simulink model "IFFT64K_2D"  (R2023b)
settings: Solver=VariableStepAuto  StartTime=0.0  StopTime=simtime  RelTol=1e-3
PostLoadFcn:
  | samp_rate = 2e9;
  | fft_sz = 65536;
  | chirp_rate = 200e6 / 1e-3;
  | tone_freq = 20e6;
  | input_bits = 12;
  | align_delay = 3 * fft_sz;
  | buff_init = complex(int32(zeros(256,1)));
  | NSTREAM = 5;
  | simtime = 2.5e-4;
undefined symbols (not defined in the file): S, vsva2197, xcvc1902
libraries: aieBasic x30, aieUtilities x15, hlsBasic x1, dspxfrm3 x1, dspsrcs4 x1, vmcUtilities x1
(part 1 of 2)
settings Model: Creator=rbuz  LastModifiedBy=robg
settings DebuggingCC: UnconnectedInputMsg=warning  UnconnectedOutputMsg=warning  UnconnectedLineMsg=warning
settings ModelReferenceCC: EnableRefExpFcnMdlSchedulingChecks=on
settings RTWCC: DLArmComputeVersion=19.05

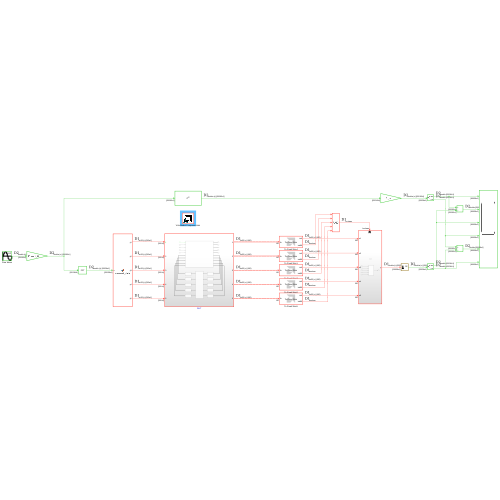
[thumbnail: Simulink's stored preview of the top-level diagram]
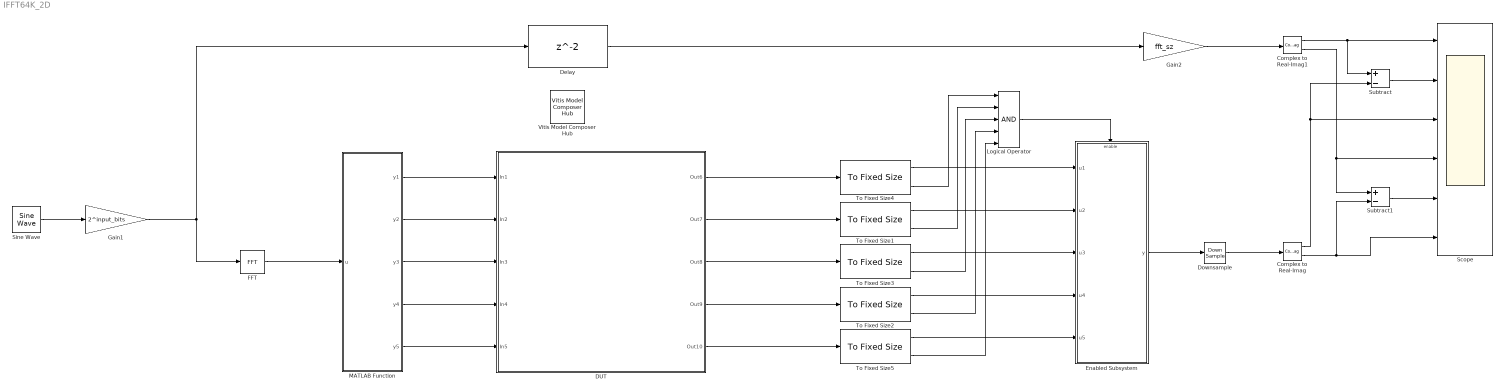
== system IFFT64K_2D ==
  Complex to Real-Imag : ComplexToRealImag
  Complex to Real-Imag1 : ComplexToRealImag
  DUT : Subsystem
  Delay : Delay
  Downsample : DownSample  N=52  RateOptions=Allow multirate processing
  Enabled Subsystem : Subsystem  TreatAsAtomicUnit=on
  FFT : dspxfrm3/FFT  FFTImplementation=Auto  CompMethod=Table lookup  TableOpt=NEW  TableOptActive=Speed  BitRevOrder=off  Normalize=off  InheritFFTLength=off  FFTLength=fft_sz  WrapInput=off  roundingMode=Floor  overflowMode=off  firstCoeffDataTypeStr=Inherit: Same word length as input  firstCoeffLastDataTypeStr=Inherit: Same word length as input  outputMin=[]  outputMax=[]
  Gain1 : Gain  Gain=2^input_bits
  Gain2 : Gain  Gain=fft_sz
  Logical Operator : Logic  Inputs=5  AllPortsSameDT=off  OutDataTypeStr=boolean
  MATLAB Function : MATLAB Function  TreatAsAtomicUnit=on  SystemSampleTime=fft_sz / (52 * samp_rate)
  Scope : Scope  NumInputPorts=6
  Sine Wave : dspsrcs4/Sine Wave  Amplitude=1  Frequency=tone_freq  Phase=0  SampleMode=Discrete  OutComplex=Complex  CompMethod=Trigonometric fcn  TableSize=Speed  SampleTime=1 / samp_rate  SamplesPerFrame=fft_sz  ResetState=Restart at time zero  OutputFrames=off  dataType=double  wordLen=16  udDataType=sfix(16)  fracBitsMode=Best precision  numFracBits=15  OutDataTypeStr=double  LastOutDataTypeStr=double
  Subtract : Sum  Inputs=+-
  Subtract1 : Sum  Inputs=+-
  To Fixed Size{1..5} (5 alike) : aieUtilities/To Fixed Size  Mode=Produce a valid output signal  OutputSize=Inherit: Same as input  CopyMethod=Buffer samples to form output  HasStatusOutput=on
  Vitis Model Composer Hub : vmcUtilities/Vitis Model Composer Hub  Tag=genX  CodeGeneration=off  SubsystemName=DUT  DUTSubsystemName=DUT  CompilationType=VitisCompilation  SubsystemType=DUTNode  ExportTypeV2=Graph Code  AIEArrayConfig=Use entire AIE array  StartColumn=20  NumberOfColumns=10  TargetDirectory=./code  exportDesign=on  analyzeDesign=off  validateDesignOnHw=off  ExportType=Vitis Subsystem  IpVendor=xilinx.com  IpLibrary=hls  IpName=ifft_transpose  IpVersion=1.0  IpHWLanguage=Verilog  AieCompilerOptions={}  AieSimulatorOptions={}  CreateTestbench=off  TestbenchStackSize=10  RunRtlSim=off  RunCSim=off  RunAieSim=on  AieSimTimeout=50000  RunAieSimProfiling=off  LaunchVitisAnalyzer=off  PlotOutput=off  RunX86Sim=off  X86SimTimeout=10  GenHwImage=off  GenLibadfXo=on  GenHwValidationCode=on  PlatformType=Specify Platform  Platform=/proj/xbuilds/SWIP/2024.2_1110_1447/installs/lin64/Vitis/2024.2/base_platforms/xilinx_vck190_base_202420_1/xilinx_vck190_base_202420_1.xpfm  HwSystemType=Baremetal  HwValidationTarget=hw_emu  ProjDevice=Versal VCK190 Evaluation Platform (xcvc1902-vsva2197-2MP-e-S)  ProjDevicePart=xcvc1902-vsva2197-2MP-e-S  AIEType=AIE  SamplePeriod=-1  ClockFrequency=200  DataPathParallelism=1  xilinxfamily=versalaicore  part=xcvc1902  speed=-2MP-e-S  package=vsva2197  directory=./netlist  testbench=off  incr_netlist=off  synthesis_tool=Vivado  clock_wrapper=Clock Enables  dbl_ovrd=According to Block Masks  dcm_input_clock_period=10  sysclk_period=10  simulink_period=1  eval_field=0  IPInfoJsonString="{\"DUTSubsystemName\":\"DUT\",\"HLSKernel\":{\"SubsystemName\":\"ifft_transpose\",\"FpgaClockFreq\":\"200\",\"IPName\":\"ifft_transpose\",\"IPLibrary\":\"hls\",\"TargetDirectory\":\"./code\",\"FreqHz\":\"200000000\",\"KernelFunction\":\"ifft_transpose_wrapper\"},\"SubsystemTag\":\"DUTNode\",\"AIESubsystem\":{\"SubsystemName\":\"AIE\",\"TargetDirectory\":\"./code\",\"AIEArrayConfig\":\"Use entire AIE array\",\"StartColumn\":\"20\",\"NumberOfColumns\":\"10\"}}"  LogFileName=/group/xcoswmktg2/robg/git/vmc_examples/Vitis_Model_Composer/Tutorials/AIE-PL/Export_to_Vitis/code/model_composer.log  NThreads=4  IPConfigFile=/tmp/vmctmp-robg/11175/ipconfig.json
  wires:
  Gain1/1 -> FFT/1, Delay/1
  Sine Wave/1 -> Gain1/1
  FFT/1 -> MATLAB Function/1(u)
  MATLAB Function/1(y1) -> DUT/1(In1)
  To Fixed Size4/1 -> Enabled Subsystem/1(u1)
  Enabled Subsystem/1(y) -> Downsample/1
  Subtract/1 -> Scope/2
  Subtract1/1 -> Scope/5
  Delay/1 -> Gain2/1
  Complex to Real-Imag1/1 -> Scope/1, Subtract/1
  Complex to Real-Imag1/2 -> Scope/4, Subtract1/1
  Complex to Real-Imag/1 -> Scope/3, Subtract/2
  Complex to Real-Imag/2 -> Subtract1/2, Scope/6
  Gain2/1 -> Complex to Real-Imag1/1
  MATLAB Function/2(y2) -> DUT/2(In2)
  MATLAB Function/3(y3) -> DUT/3(In3)
  MATLAB Function/4(y4) -> DUT/4(In4)
  MATLAB Function/5(y5) -> DUT/5(In5)
  To Fixed Size1/1 -> Enabled Subsystem/2(u2)
  To Fixed Size3/1 -> Enabled Subsystem/3(u3)
  To Fixed Size2/1 -> Enabled Subsystem/4(u4)
  To Fixed Size5/1 -> Enabled Subsystem/5(u5)
  Logical Operator/1 -> Enabled Subsystem/Enable
  To Fixed Size4/2 -> Logical Operator/1
  To Fixed Size1/2 -> Logical Operator/2
  To Fixed Size3/2 -> Logical Operator/3
  To Fixed Size2/2 -> Logical Operator/4
  To Fixed Size5/2 -> Logical Operator/5
  DUT/1(Out6) -> To Fixed Size4/1
  DUT/2(Out7) -> To Fixed Size1/1
  DUT/3(Out8) -> To Fixed Size3/1
  DUT/4(Out9) -> To Fixed Size2/1
  DUT/5(Out10) -> To Fixed Size5/1
  Downsample/1 -> Complex to Real-Imag/1

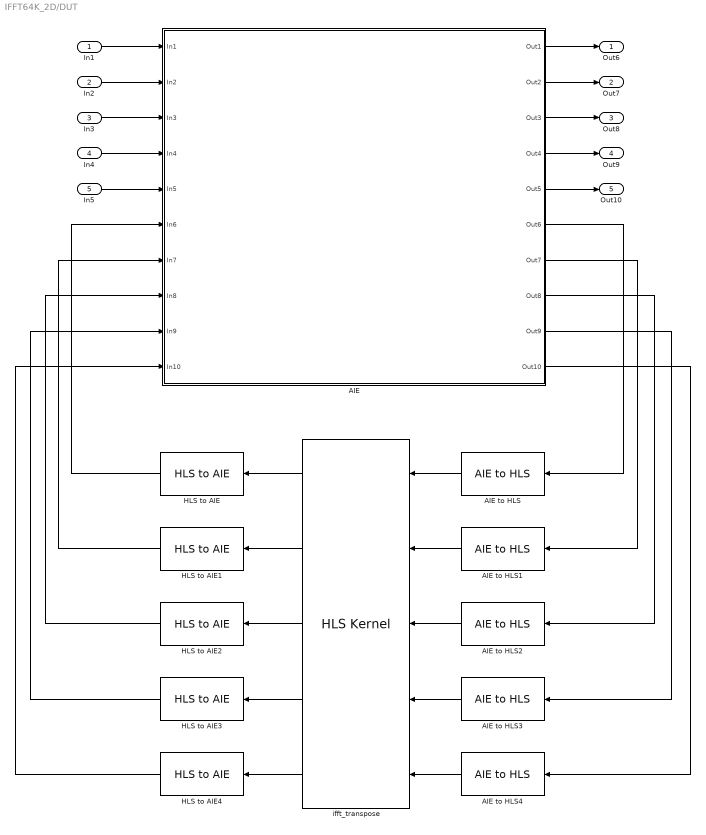
== system IFFT64K_2D/DUT ==
  In1 : Inport
  In2 : Inport  Port=2
  In3 : Inport  Port=3
  In4 : Inport  Port=4
  In5 : Inport  Port=5
  AIE : Subsystem
  AIE to HLS{,1..4} (5 alike) : aieUtilities/AIE to HLS  OutputType=ufix128  OutputSize=130
  HLS to AIE{,1..4} (5 alike) : aieUtilities/HLS to AIE  OutputType=cint32  OutputSize=260
  ifft_transpose : hlsBasic/HLS Kernel  PortNames={'return'; 'sig_0_i'; 'sig_1_i'; 'sig_2_i'; 'sig_3_i'; 'sig_4_i'; 'sig_0_o'; 'sig_1_o'; 'sig_2_o'; 'sig_3_o'; 'sig_4_o'}  PortSerializedTypes={'{Bv}'; '{R{Thls::stream{2{t{Tap_uint{1{t{}128}}}}{t{}0}}}}'; '{R{Thls::stream{2{t{Tap_uint{1{t{}128}}}}{t{}0}}}}'; '{R{Thls::stream{2{t{Tap_uint{1{t{}128}}}}{t{}0}}}}'; '{R{Thls::stream{2{t{Tap_uint{1{t{}128}}}}{t{}0}}}}'; '{R{Thls::stream{2{t{Tap_uint{1{t{}128}}}}{t{}0}}}}'; '{R{Thls::stream{2{t{Tap_uint{1{t{}128}}}}{t{}0}}}}'; '{R{Thls::stream{2{t{Tap_uint{1{t{}128}}}}{t{}0}}}}'; '{R{Thls::stream{2{t{Tap_uint{1{t{}128}}}}{t{}0}}}}'; '{R{Thls::stream{2{t{Tap_uint{1{t{}128}}}}{t{}0}}}}'; '{R{Thls::stream{2{t{Tap_uint{1{t{}128}}}}{t{}0}}}}'}  FunctionTemplateSpecKind=none  FunctionTemplateParamNames={}  FunctionTemplateParamKinds={}  FunctionTemplateParamTypes={}  FunctionTemplateParamValues={}  PortSynchronicities={'auto'; 'auto'; 'auto'; 'auto'; 'auto'; 'auto'; 'auto'; 'auto'; 'auto'; 'auto'}  PortSignalSizes={0.000000000000000000e+00; 0.000000000000000000e+00; 0.000000000000000000e+00; 0.000000000000000000e+00; 0.000000000000000000e+00; 1.300000000000000000e+02; 1.300000000000000000e+02; 1.300000000000000000e+02; 1.300000000000000000e+02; 1.300000000000000000e+02}  PortParameterValues={}  FunctionTemplateParams={}  FunctionTemplateParamsEnables={}  FunctionTemplateParamsVisible=off  FunctionDeclTypeOptions=C[1 1]@t7@<empty>  PortAttributesTable={ 'Input', 'sig_0_i', 'hls::stream< ap_uint< 128 >, 0 > &', '', ''; 'Input', 'sig_1_i', 'hls::stream< ap_uint< 128 >, 0 > &', '', ''; 'Input', 'sig_2_i', 'hls::stream< ap_uint< 128 >, 0 > &', '', ''; 'Input', 'sig_3_i', 'hls::stream< ap_uint< 128 >, 0 > &', '', ''; 'Input', 'sig_4_i', 'hls::stream< ap_uint< 128 >, 0 > &', '', ''; 'Output', 'sig_0_o', 'hls::stream< ap_uint< 128 >, 0 > &', '', '130'; 'Output', 'sig_1_o', 'hls::stream< ap_uint< 128 >, 0 > &', '', '130'; 'Output', 'sig_2_o', 'hls::stream< ap_uint< 128 >, 0 > &', '', '130'; 'Output', 'sig_3_o', 'hls::stream< ap_uint< 128 >, 0 > &', '', '130'; 'Output', 'sig_4_o', 'hls::stream< ap_uint< 128 >, 0 > &', '', '130' }  PortAttributesEnablement={'off', 'off', 'off', 'off', 'off';'off', 'off', 'off', 'off', 'off';'off', 'off', 'off', 'off', 'off';'off', 'off', 'off', 'off', 'off';'off', 'off', 'off', 'off', 'off';'off', 'off', 'off', 'off', 'on';'off', 'off', 'off', 'off', 'on';'off', 'off', 'off', 'off', 'on';'off', 'off', 'off', 'off', 'on';'off', 'off', 'off', 'off', 'on'}  PortParametersTable={}  SampleTime=-1  PortDirectionTable={ 'sig_0_i', 'hls::stream< ap_uint< 128 >, 0 > &', 'Input', 'Port'; 'sig_1_i', 'hls::stream< ap_uint< 128 >, 0 > &', 'Input', 'Port'; 'sig_2_i', 'hls::stream< ap_uint< 128 >, 0 > &', 'Input', 'Port'; 'sig_3_i', 'hls::stream< ap_uint< 128 >, 0 > &', 'Input', 'Port'; 'sig_4_i', 'hls::stream< ap_uint< 128 >, 0 > &', 'Input', 'Port'; 'sig_0_o', 'hls::stream< ap_uint< 128 >, 0 > &', 'Output', 'Port'; 'sig_1_o', 'hls::stream< ap_uint< 128 >, 0 > &', 'Output', 'Port'; 'sig_2_o', 'hls::stream< ap_uint< 128 >, 0 > &', 'Output', 'Port'; 'sig_3_o', 'hls::stream< ap_uint< 128 >, 0 > &', 'Output', 'Port'; 'sig_4_o', 'hls::stream< ap_uint< 128 >, 0 > &', 'Output', 'Port' }  PortDirectionTabVisible=on  ArgDirections={1.000000000000000000e+00; 1.000000000000000000e+00; 1.000000000000000000e+00; 1.000000000000000000e+00; 1.000000000000000000e+00; 2.000000000000000000e+00; 2.000000000000000000e+00; 2.000000000000000000e+00; 2.000000000000000000e+00; 2.000000000000000000e+00}  ArgInterfaceTypes={1.000000000000000000e+00; 1.000000000000000000e+00; 1.000000000000000000e+00; 1.000000000000000000e+00; 1.000000000000000000e+00; 1.000000000000000000e+00; 1.000000000000000000e+00; 1.000000000000000000e+00; 1.000000000000000000e+00; 1.000000000000000000e+00}  FunctionIndex=1  FormalArgDecls={'hls::stream< ap_uint< 128 >, 0 > & sig_0_i', 'hls::stream< ap_uint< 128 >, 0 > & sig_1_i', 'hls::stream< ap_uint< 128 >, 0 > & sig_2_i', 'hls::stream< ap_uint< 128 >, 0 > & sig_3_i', 'hls::stream< ap_uint< 128 >, 0 > & sig_4_i', 'hls::stream< ap_uint< 128 >, 0 > & sig_0_o', 'hls::stream< ap_uint< 128 >, 0 > & sig_1_o', 'hls::stream< ap_uint< 128 >, 0 > & sig_2_o', 'hls::stream< ap_uint< 128 >, 0 > & sig_3_o', 'hls::stream< ap_uint< 128 >, 0 > & sig_4_o'}  SimLibPath=''  FunctionTabVisible=on  FunctionDescription=void ifft_transpose_wrapper(hls::stream< ap_uint< 128 >, 0 > & sig_0_i, hls::stream< ap_uint< 128 >, 0 > & sig_1_i, hls::stream< ap_uint< 128 >, 0 > & sig_2_i, hls::stream< ap_uint< 128 >, 0 > & sig_3_i, hls::stream< ap_uint< 128 >, 0 > & sig_4_i, hls::stream< ap_uint< 128 >, 0 > & sig_0_o, hls::stream< ap_uint< 128 >, 0 > & sig_1_o, hls::stream< ap_uint< 128 >, 0 > & sig_2_o, hls::stream< ap_uint< 128 >, 0 > & sig_3_o, hls::stream< ap_uint< 128 >, 0 > & sig_4_o)  blockJsonConstraints=[]  deprecateConstraints=0  KernelHeaderFile=hls_src/ifft_transpose_vmc.h  KernelFunction=ifft_transpose_wrapper  KernelFunctionSelect=<empty>  KernelSourceFile=hls_src/ifft_transpose_vmc.cpp  KernelSearchPaths={}  PreProcOptions={}
  Out6 : Outport
  Out7 : Outport  Port=2
  Out8 : Outport  Port=3
  Out9 : Outport  Port=4
  Out10 : Outport  Port=5
  wires:
  HLS to AIE2/1 -> AIE/8(In8)
  AIE to HLS2/1 -> ifft_transpose/3
  HLS to AIE/1 -> AIE/6(In6)
  AIE to HLS/1 -> ifft_transpose/1
  ifft_transpose/2 -> HLS to AIE1/1
  ifft_transpose/3 -> HLS to AIE2/1
  ifft_transpose/5 -> HLS to AIE4/1
  HLS to AIE1/1 -> AIE/7(In7)
  AIE/9(Out9) -> AIE to HLS3/1
  ifft_transpose/4 -> HLS to AIE3/1
  AIE to HLS3/1 -> ifft_transpose/4
  ifft_transpose/1 -> HLS to AIE/1
  HLS to AIE3/1 -> AIE/9(In9)
  HLS to AIE4/1 -> AIE/10(In10)
  AIE/6(Out6) -> AIE to HLS/1
  AIE/7(Out7) -> AIE to HLS1/1
  AIE/8(Out8) -> AIE to HLS2/1
  AIE/10(Out10) -> AIE to HLS4/1
  AIE to HLS4/1 -> ifft_transpose/5
  AIE to HLS1/1 -> ifft_transpose/2
  In1/1 -> AIE/1(In1)
  In2/1 -> AIE/2(In2)
  In3/1 -> AIE/3(In3)
  In4/1 -> AIE/4(In4)
  In5/1 -> AIE/5(In5)
  AIE/1(Out1) -> Out6/1
  AIE/2(Out2) -> Out7/1
  AIE/3(Out3) -> Out8/1
  AIE/4(Out4) -> Out9/1
  AIE/5(Out5) -> Out10/1

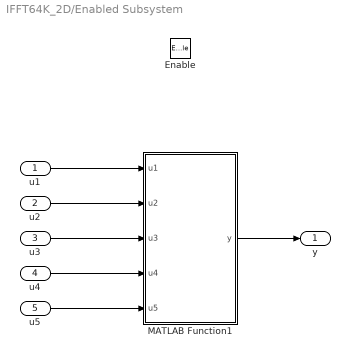
== system IFFT64K_2D/Enabled Subsystem ==
  u1 : Inport
  u2 : Inport  Port=2
  u3 : Inport  Port=3
  u4 : Inport  Port=4
  u5 : Inport  Port=5
  Enable : EnablePort
  MATLAB Function1 : MATLAB Function  TreatAsAtomicUnit=on
  y : Outport
  wires:
  MATLAB Function1/1(y) -> y/1
  u1/1 -> MATLAB Function1/1(u1)
  u2/1 -> MATLAB Function1/2(u2)
  u3/1 -> MATLAB Function1/3(u3)
  u4/1 -> MATLAB Function1/4(u4)
  u5/1 -> MATLAB Function1/5(u5)

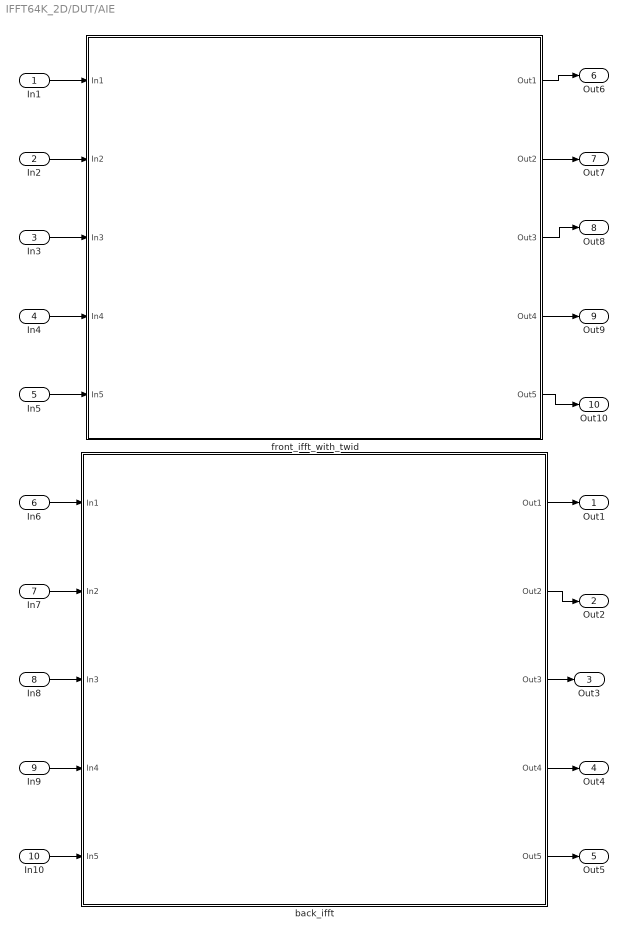
== system IFFT64K_2D/DUT/AIE ==
  In1 : Inport
  In2 : Inport  Port=2
  In3 : Inport  Port=3
  In4 : Inport  Port=4
  In5 : Inport  Port=5
  In6 : Inport  Port=6
  In7 : Inport  Port=7
  In8 : Inport  Port=8
  In9 : Inport  Port=9
  In10 : Inport  Port=10
  back_ifft : Subsystem
  front_ifft_with_twid : Subsystem
  Out1 : Outport
  Out2 : Outport  Port=2
  Out3 : Outport  Port=3
  Out4 : Outport  Port=4
  Out5 : Outport  Port=5
  Out6 : Outport  Port=6
  Out7 : Outport  Port=7
  Out8 : Outport  Port=8
  Out9 : Outport  Port=9
  Out10 : Outport  Port=10
  wires:
  front_ifft_with_twid/1(Out1) -> Out6/1
  front_ifft_with_twid/5(Out5) -> Out10/1
  In1/1 -> front_ifft_with_twid/1(In1)
  In2/1 -> front_ifft_with_twid/2(In2)
  In5/1 -> front_ifft_with_twid/5(In5)
  In4/1 -> front_ifft_with_twid/4(In4)
  In3/1 -> front_ifft_with_twid/3(In3)
  front_ifft_with_twid/2(Out2) -> Out7/1
  front_ifft_with_twid/3(Out3) -> Out8/1
  front_ifft_with_twid/4(Out4) -> Out9/1
  In6/1 -> back_ifft/1(In1)
  In7/1 -> back_ifft/2(In2)
  In8/1 -> back_ifft/3(In3)
  In9/1 -> back_ifft/4(In4)
  In10/1 -> back_ifft/5(In5)
  back_ifft/1(Out1) -> Out1/1
  back_ifft/3(Out3) -> Out3/1
  back_ifft/2(Out2) -> Out2/1
  back_ifft/5(Out5) -> Out5/1
  back_ifft/4(Out4) -> Out4/1

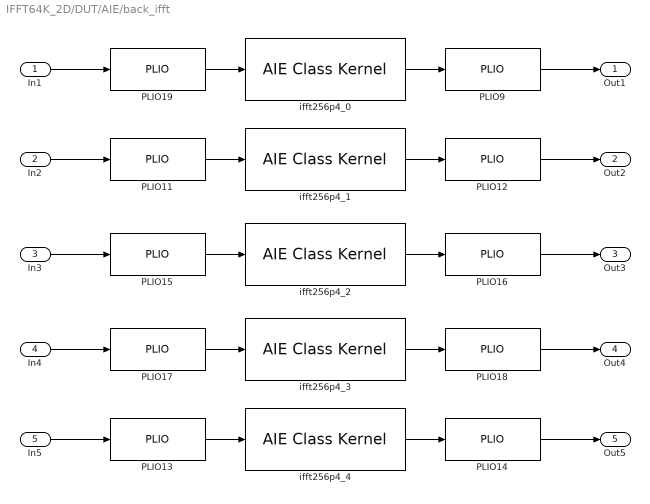
== system IFFT64K_2D/DUT/AIE/back_ifft ==
  In1 : Inport
  In2 : Inport  Port=2
  In3 : Inport  Port=3
  In4 : Inport  Port=4
  In5 : Inport  Port=5
  PLIO{9,11..19} (10 alike) : aieBasic/PLIO  PlioWidth=64  PlioFreqSpec=off  PlioFreq=250  ColLocation=0  channel=0  blockJsonConstraints=[]  deprecateConstraints=0
  ifft256p4_0 : aieBasic/AIE Class Kernel  KernelAllAttrs=|  PortNames={'sig_i'; 'sig_o'}  PortSerializedTypes={'{Q2{R{Tadf::input_buffer{2{t{Scint32}}{t{Tadf::extents{1{t{}260}}}}}}}}'; '{Q2{R{Tadf::output_buffer{2{t{Scint32}}{t{Tadf::extents{1{t{}260}}}}}}}}'}  PortWindowSizes={2.600000000000000000e+02; 2.600000000000000000e+02}  PortWindowMargins={0.000000000000000000e+00; 0.000000000000000000e+00}  PortSynchronicities={'sync', 'sync'}  PortSignalSizes={0.000000000000000000e+00; 0.000000000000000000e+00}  ClassTemplateSpecKind=none  ClassTemplateParamNames={}  ClassTemplateParamKinds={}  ClassTemplateParamTypes={}  ClassTemplateParamValues={}  ClassCtorParamNames={'tbuff_i'}  ClassCtorParamSerializedTypes={'{R{C{Scint32}256}}'}  ClassCtorParamValues={'[0;0;0;0;0;0;0;0;0;0;0;0;0;0;0;0;0;0;0;0;0;0;0;0;0;0;0;0;0;0;0;0;0;0;0;0;0;0;0;0;0;0;0;0;0;0;0;0;0;0;0;0;0;0;0;0;0;0;0;0;0;0;0;0;0;0;0;0;0;0;0;0;0;0;0;0;0;0;0;0;0;0;0;0;0;0;0;0;0;0;0;0;0;0;0;0;0;0;0;0;0;0;0;0;0;0;0;0;0;0;0;0;0;0;0;0;0;0;0;0;0;0;0;0;0;0;0;0;0;0;0;0;0;0;0;0;0;0;0;0;0;0;0;0;0;0;0;0;0;0;0;0;0;0;0;0;0;0;0;0;0;0;0;0;0;0;0;0;0;0;0;0;0;0;0;0;0;0;0;0;0;0;0;0;0;0;0;0;0;0;0;0;0;0;0;0;0;0;0;0;0;0;0;0;0;0;0;0;0;0;0;0;0;0;0;0;0;0;0;0;0;0;0;0;0;0;0;0;0;0;0;0;0;0;0;0;0;0;0;0;0;0;0;0;0;0;0;0;0;0;0;0;0;0;0;0]'}  ClassIndex=1  ClassCtorIndex=1  ClassTabVisible=on  ClassTemplateParamsVisible=off  ClassCtorDeclVisible=on  ClassCtorParamsVisible=on  FunctionTabVisible=on  FunctionDecl=|  PortAttrs={ 'input', 'sig_i', 'adf::input_buffer< cint32, adf::extents< 260 > > & restrict', '260', '0', 'sync', ''; 'output', 'sig_o', 'adf::output_buffer< cint32, adf::extents< 260 > > & restrict', '260', '', 'sync', '' }  PortAttrsEnables={'off', 'off', 'off', 'off', 'off', 'off', 'off';'off', 'off', 'off', 'off', 'off', 'off', 'off'}  SampleTime=-1  ClassDeclTypeOptions=C[1 1]@t16@class ifft256p4;  ClassDecl=class ifft256p4;  ClassTemplateParams={}  ClassTemplateParamsEnables={}  ClassCtorDeclTypeOptions=C[1 1]@t39@ifft256p4(cint32 ( & tbuff_i ) [ 256 ])  ClassCtorDecl=ifft256p4(cint32 ( & tbuff_i ) [ 256 ])  ClassCtorParams={ 'tbuff_i', 'cint32 ( &) [ 256 ]', 'buff_init' }  KernelHeaderFile=aie_src/ifft256p4.h  KernelClassName=ifft256p4  KernelFunction=run  KernelSourceFile=aie_src/ifft256p4.cpp  KernelSearchPaths={}  PreProcOptions={}  blockJsonConstraints=[]
      KernelAllAttrs=|
      | s[12;12;9;9;19;14;21;23;21;23;24;21;15;17;12;24;26;26;26;27;28;9;21;23;23;23;24;25;14;19;19;29]@FunctionNameDeclFileNamePortNamesPortTypesPortSerializedTypesPortDirectionsPortWindowSizeEnablesPortWindowMarginEnablesPortBufferSizeEnablesPortBufferMarginEnablesPortSynchronicityEnablesPortSignalSizeEnablesPortBufferSizesPortBufferMarginsFunctionDeclFunctionTemplateSpecKindFunctionTemplateParamNamesFunctionTemplateParamKindsFunctionTemplateParamTypesFunctionTemplateParamValuesFunctionTemplateParamEnablesClassDeclClassTemplateSpecKindClassTemplateParamNamesClassTemplateParamKindsClassTemplateParamTypesClassTemplateParamValuesClassTemplateParamEnablesClassCtorDeclsClassCtorParamNamesClassCtorParamTypesClassCtorParamSerializedTypes[1 1]@C[32 1]@t3@runt29@../../aie_src/ifft256p4_vmc.hC[2 1]@t5@sig_it5@sig_oC[2 1]@t59@adf::input_buffer< cint32, adf::extents< 260 > > & restrictt60@adf::output_buffer< cint32, adf::extents< 260 > > & restrictC[2 1]@t71@{Q2{R{Tadf::input_buffer{2{t{Scint32}}{t{Tadf::extents{1{t{}260}}}}}}}}t72@{Q2{R{Tadf::output_buffer{2{t{Scint32}}{t{Tadf::extents{1{t{}260}}}}}}}}C[2 1]@t5@inputt6@outputC[2 1]@l1@l1@C[2 1]@l1@l0@C[2 1]@l1@l1@C[2 1]@l0@l0@C[2 1]@l1@l1@C[2 1]@l0@l0@C[2 1]@t3@260t3@260C[2 1]@nnt155@void ifft256p4::
      | run(adf::input_buffer< cint32, adf::extents< 260 > > & restrict sig_i, adf::output_buffer< cint32, adf::extents< 260 > > & restrict sig_o)t4@nonee[0 1]@e[0 1]@e[0 1]@e[0 1]@e[0 1]@t16@class ifft256p4;t4@nonee[0 1]@e[0 1]@e[0 1]@e[0 1]@e[0 1]@C[1 1]@t39@ifft256p4(cint32 ( & tbuff_i ) [ 256 ])C[1 1]@C[1 1]@t7@tbuff_iC[1 1]@C[1 1]@t19@cint32 ( &) [ 256 ]C[1 1]@C[1 1]@t18@{R{C{Scint32}256}}
      FunctionDecl=|
      | void ifft256p4::
      | run(adf::input_buffer< cint32, adf::extents< 260 > > & restrict sig_i, adf::output_buffer< cint32, adf::extents< 260 > > & restrict sig_o)
  ifft256p4_1 : aieBasic/AIE Class Kernel  KernelAllAttrs=|  PortNames={'sig_i'; 'sig_o'}  PortSerializedTypes={'{Q2{R{Tadf::input_buffer{2{t{Scint32}}{t{Tadf::extents{1{t{}260}}}}}}}}'; '{Q2{R{Tadf::output_buffer{2{t{Scint32}}{t{Tadf::extents{1{t{}260}}}}}}}}'}  PortWindowSizes={2.600000000000000000e+02; 2.600000000000000000e+02}  PortWindowMargins={0.000000000000000000e+00; 0.000000000000000000e+00}  PortSynchronicities={'sync', 'sync'}  PortSignalSizes={0.000000000000000000e+00; 0.000000000000000000e+00}  ClassTemplateSpecKind=none  ClassTemplateParamNames={}  ClassTemplateParamKinds={}  ClassTemplateParamTypes={}  ClassTemplateParamValues={}  ClassCtorParamNames={'tbuff_i'}  ClassCtorParamSerializedTypes={'{R{C{Scint32}256}}'}  ClassCtorParamValues={'[0;0;0;0;0;0;0;0;0;0;0;0;0;0;0;0;0;0;0;0;0;0;0;0;0;0;0;0;0;0;0;0;0;0;0;0;0;0;0;0;0;0;0;0;0;0;0;0;0;0;0;0;0;0;0;0;0;0;0;0;0;0;0;0;0;0;0;0;0;0;0;0;0;0;0;0;0;0;0;0;0;0;0;0;0;0;0;0;0;0;0;0;0;0;0;0;0;0;0;0;0;0;0;0;0;0;0;0;0;0;0;0;0;0;0;0;0;0;0;0;0;0;0;0;0;0;0;0;0;0;0;0;0;0;0;0;0;0;0;0;0;0;0;0;0;0;0;0;0;0;0;0;0;0;0;0;0;0;0;0;0;0;0;0;0;0;0;0;0;0;0;0;0;0;0;0;0;0;0;0;0;0;0;0;0;0;0;0;0;0;0;0;0;0;0;0;0;0;0;0;0;0;0;0;0;0;0;0;0;0;0;0;0;0;0;0;0;0;0;0;0;0;0;0;0;0;0;0;0;0;0;0;0;0;0;0;0;0;0;0;0;0;0;0;0;0;0;0;0;0;0;0;0;0;0;0]'}  ClassIndex=1  ClassCtorIndex=1  ClassTabVisible=on  ClassTemplateParamsVisible=off  ClassCtorDeclVisible=on  ClassCtorParamsVisible=on  FunctionTabVisible=on  FunctionDecl=|  PortAttrs={ 'input', 'sig_i', 'adf::input_buffer< cint32, adf::extents< 260 > > & restrict', '260', '0', 'sync', ''; 'output', 'sig_o', 'adf::output_buffer< cint32, adf::extents< 260 > > & restrict', '260', '', 'sync', '' }  PortAttrsEnables={'off', 'off', 'off', 'off', 'off', 'off', 'off';'off', 'off', 'off', 'off', 'off', 'off', 'off'}  SampleTime=-1  ClassDeclTypeOptions=C[1 1]@t16@class ifft256p4;  ClassDecl=class ifft256p4;  ClassTemplateParams={}  ClassTemplateParamsEnables={}  ClassCtorDeclTypeOptions=C[1 1]@t39@ifft256p4(cint32 ( & tbuff_i ) [ 256 ])  ClassCtorDecl=ifft256p4(cint32 ( & tbuff_i ) [ 256 ])  ClassCtorParams={ 'tbuff_i', 'cint32 ( &) [ 256 ]', 'buff_init' }  KernelHeaderFile=aie_src/ifft256p4.h  KernelClassName=ifft256p4  KernelFunction=run  KernelSourceFile=aie_src/ifft256p4.cpp  KernelSearchPaths={}  PreProcOptions={}  blockJsonConstraints=[]
      KernelAllAttrs=|
      | s[12;12;9;9;19;14;21;23;21;23;24;21;15;17;12;24;26;26;26;27;28;9;21;23;23;23;24;25;14;19;19;29]@FunctionNameDeclFileNamePortNamesPortTypesPortSerializedTypesPortDirectionsPortWindowSizeEnablesPortWindowMarginEnablesPortBufferSizeEnablesPortBufferMarginEnablesPortSynchronicityEnablesPortSignalSizeEnablesPortBufferSizesPortBufferMarginsFunctionDeclFunctionTemplateSpecKindFunctionTemplateParamNamesFunctionTemplateParamKindsFunctionTemplateParamTypesFunctionTemplateParamValuesFunctionTemplateParamEnablesClassDeclClassTemplateSpecKindClassTemplateParamNamesClassTemplateParamKindsClassTemplateParamTypesClassTemplateParamValuesClassTemplateParamEnablesClassCtorDeclsClassCtorParamNamesClassCtorParamTypesClassCtorParamSerializedTypes[1 1]@C[32 1]@t3@runt29@../../aie_src/ifft256p4_vmc.hC[2 1]@t5@sig_it5@sig_oC[2 1]@t59@adf::input_buffer< cint32, adf::extents< 260 > > & restrictt60@adf::output_buffer< cint32, adf::extents< 260 > > & restrictC[2 1]@t71@{Q2{R{Tadf::input_buffer{2{t{Scint32}}{t{Tadf::extents{1{t{}260}}}}}}}}t72@{Q2{R{Tadf::output_buffer{2{t{Scint32}}{t{Tadf::extents{1{t{}260}}}}}}}}C[2 1]@t5@inputt6@outputC[2 1]@l1@l1@C[2 1]@l1@l0@C[2 1]@l1@l1@C[2 1]@l0@l0@C[2 1]@l1@l1@C[2 1]@l0@l0@C[2 1]@t3@260t3@260C[2 1]@nnt155@void ifft256p4::
      | run(adf::input_buffer< cint32, adf::extents< 260 > > & restrict sig_i, adf::output_buffer< cint32, adf::extents< 260 > > & restrict sig_o)t4@nonee[0 1]@e[0 1]@e[0 1]@e[0 1]@e[0 1]@t16@class ifft256p4;t4@nonee[0 1]@e[0 1]@e[0 1]@e[0 1]@e[0 1]@C[1 1]@t39@ifft256p4(cint32 ( & tbuff_i ) [ 256 ])C[1 1]@C[1 1]@t7@tbuff_iC[1 1]@C[1 1]@t19@cint32 ( &) [ 256 ]C[1 1]@C[1 1]@t18@{R{C{Scint32}256}}
      FunctionDecl=|
      | void ifft256p4::
      | run(adf::input_buffer< cint32, adf::extents< 260 > > & restrict sig_i, adf::output_buffer< cint32, adf::extents< 260 > > & restrict sig_o)
  ifft256p4_2 : aieBasic/AIE Class Kernel  KernelAllAttrs=|  PortNames={'sig_i'; 'sig_o'}  PortSerializedTypes={'{Q2{R{Tadf::input_buffer{2{t{Scint32}}{t{Tadf::extents{1{t{}260}}}}}}}}'; '{Q2{R{Tadf::output_buffer{2{t{Scint32}}{t{Tadf::extents{1{t{}260}}}}}}}}'}  PortWindowSizes={2.600000000000000000e+02; 2.600000000000000000e+02}  PortWindowMargins={0.000000000000000000e+00; 0.000000000000000000e+00}  PortSynchronicities={'sync', 'sync'}  PortSignalSizes={0.000000000000000000e+00; 0.000000000000000000e+00}  ClassTemplateSpecKind=none  ClassTemplateParamNames={}  ClassTemplateParamKinds={}  ClassTemplateParamTypes={}  ClassTemplateParamValues={}  ClassCtorParamNames={'tbuff_i'}  ClassCtorParamSerializedTypes={'{R{C{Scint32}256}}'}  ClassCtorParamValues={'[0;0;0;0;0;0;0;0;0;0;0;0;0;0;0;0;0;0;0;0;0;0;0;0;0;0;0;0;0;0;0;0;0;0;0;0;0;0;0;0;0;0;0;0;0;0;0;0;0;0;0;0;0;0;0;0;0;0;0;0;0;0;0;0;0;0;0;0;0;0;0;0;0;0;0;0;0;0;0;0;0;0;0;0;0;0;0;0;0;0;0;0;0;0;0;0;0;0;0;0;0;0;0;0;0;0;0;0;0;0;0;0;0;0;0;0;0;0;0;0;0;0;0;0;0;0;0;0;0;0;0;0;0;0;0;0;0;0;0;0;0;0;0;0;0;0;0;0;0;0;0;0;0;0;0;0;0;0;0;0;0;0;0;0;0;0;0;0;0;0;0;0;0;0;0;0;0;0;0;0;0;0;0;0;0;0;0;0;0;0;0;0;0;0;0;0;0;0;0;0;0;0;0;0;0;0;0;0;0;0;0;0;0;0;0;0;0;0;0;0;0;0;0;0;0;0;0;0;0;0;0;0;0;0;0;0;0;0;0;0;0;0;0;0;0;0;0;0;0;0;0;0;0;0;0;0]'}  ClassIndex=1  ClassCtorIndex=1  ClassTabVisible=on  ClassTemplateParamsVisible=off  ClassCtorDeclVisible=on  ClassCtorParamsVisible=on  FunctionTabVisible=on  FunctionDecl=|  PortAttrs={ 'input', 'sig_i', 'adf::input_buffer< cint32, adf::extents< 260 > > & restrict', '260', '0', 'sync', ''; 'output', 'sig_o', 'adf::output_buffer< cint32, adf::extents< 260 > > & restrict', '260', '', 'sync', '' }  PortAttrsEnables={'off', 'off', 'off', 'off', 'off', 'off', 'off';'off', 'off', 'off', 'off', 'off', 'off', 'off'}  SampleTime=-1  ClassDeclTypeOptions=C[1 1]@t16@class ifft256p4;  ClassDecl=class ifft256p4;  ClassTemplateParams={}  ClassTemplateParamsEnables={}  ClassCtorDeclTypeOptions=C[1 1]@t39@ifft256p4(cint32 ( & tbuff_i ) [ 256 ])  ClassCtorDecl=ifft256p4(cint32 ( & tbuff_i ) [ 256 ])  ClassCtorParams={ 'tbuff_i', 'cint32 ( &) [ 256 ]', 'buff_init' }  KernelHeaderFile=aie_src/ifft256p4.h  KernelClassName=ifft256p4  KernelFunction=run  KernelSourceFile=aie_src/ifft256p4.cpp  KernelSearchPaths={}  PreProcOptions={}  blockJsonConstraints=[]
      KernelAllAttrs=|
      | s[12;12;9;9;19;14;21;23;21;23;24;21;15;17;12;24;26;26;26;27;28;9;21;23;23;23;24;25;14;19;19;29]@FunctionNameDeclFileNamePortNamesPortTypesPortSerializedTypesPortDirectionsPortWindowSizeEnablesPortWindowMarginEnablesPortBufferSizeEnablesPortBufferMarginEnablesPortSynchronicityEnablesPortSignalSizeEnablesPortBufferSizesPortBufferMarginsFunctionDeclFunctionTemplateSpecKindFunctionTemplateParamNamesFunctionTemplateParamKindsFunctionTemplateParamTypesFunctionTemplateParamValuesFunctionTemplateParamEnablesClassDeclClassTemplateSpecKindClassTemplateParamNamesClassTemplateParamKindsClassTemplateParamTypesClassTemplateParamValuesClassTemplateParamEnablesClassCtorDeclsClassCtorParamNamesClassCtorParamTypesClassCtorParamSerializedTypes[1 1]@C[32 1]@t3@runt29@../../aie_src/ifft256p4_vmc.hC[2 1]@t5@sig_it5@sig_oC[2 1]@t59@adf::input_buffer< cint32, adf::extents< 260 > > & restrictt60@adf::output_buffer< cint32, adf::extents< 260 > > & restrictC[2 1]@t71@{Q2{R{Tadf::input_buffer{2{t{Scint32}}{t{Tadf::extents{1{t{}260}}}}}}}}t72@{Q2{R{Tadf::output_buffer{2{t{Scint32}}{t{Tadf::extents{1{t{}260}}}}}}}}C[2 1]@t5@inputt6@outputC[2 1]@l1@l1@C[2 1]@l1@l0@C[2 1]@l1@l1@C[2 1]@l0@l0@C[2 1]@l1@l1@C[2 1]@l0@l0@C[2 1]@t3@260t3@260C[2 1]@nnt155@void ifft256p4::
      | run(adf::input_buffer< cint32, adf::extents< 260 > > & restrict sig_i, adf::output_buffer< cint32, adf::extents< 260 > > & restrict sig_o)t4@nonee[0 1]@e[0 1]@e[0 1]@e[0 1]@e[0 1]@t16@class ifft256p4;t4@nonee[0 1]@e[0 1]@e[0 1]@e[0 1]@e[0 1]@C[1 1]@t39@ifft256p4(cint32 ( & tbuff_i ) [ 256 ])C[1 1]@C[1 1]@t7@tbuff_iC[1 1]@C[1 1]@t19@cint32 ( &) [ 256 ]C[1 1]@C[1 1]@t18@{R{C{Scint32}256}}
      FunctionDecl=|
      | void ifft256p4::
      | run(adf::input_buffer< cint32, adf::extents< 260 > > & restrict sig_i, adf::output_buffer< cint32, adf::extents< 260 > > & restrict sig_o)
  ifft256p4_3 : aieBasic/AIE Class Kernel  KernelAllAttrs=|  PortNames={'sig_i'; 'sig_o'}  PortSerializedTypes={'{Q2{R{Tadf::input_buffer{2{t{Scint32}}{t{Tadf::extents{1{t{}260}}}}}}}}'; '{Q2{R{Tadf::output_buffer{2{t{Scint32}}{t{Tadf::extents{1{t{}260}}}}}}}}'}  PortWindowSizes={2.600000000000000000e+02; 2.600000000000000000e+02}  PortWindowMargins={0.000000000000000000e+00; 0.000000000000000000e+00}  PortSynchronicities={'sync', 'sync'}  PortSignalSizes={0.000000000000000000e+00; 0.000000000000000000e+00}  ClassTemplateSpecKind=none  ClassTemplateParamNames={}  ClassTemplateParamKinds={}  ClassTemplateParamTypes={}  ClassTemplateParamValues={}  ClassCtorParamNames={'tbuff_i'}  ClassCtorParamSerializedTypes={'{R{C{Scint32}256}}'}  ClassCtorParamValues={'[0;0;0;0;0;0;0;0;0;0;0;0;0;0;0;0;0;0;0;0;0;0;0;0;0;0;0;0;0;0;0;0;0;0;0;0;0;0;0;0;0;0;0;0;0;0;0;0;0;0;0;0;0;0;0;0;0;0;0;0;0;0;0;0;0;0;0;0;0;0;0;0;0;0;0;0;0;0;0;0;0;0;0;0;0;0;0;0;0;0;0;0;0;0;0;0;0;0;0;0;0;0;0;0;0;0;0;0;0;0;0;0;0;0;0;0;0;0;0;0;0;0;0;0;0;0;0;0;0;0;0;0;0;0;0;0;0;0;0;0;0;0;0;0;0;0;0;0;0;0;0;0;0;0;0;0;0;0;0;0;0;0;0;0;0;0;0;0;0;0;0;0;0;0;0;0;0;0;0;0;0;0;0;0;0;0;0;0;0;0;0;0;0;0;0;0;0;0;0;0;0;0;0;0;0;0;0;0;0;0;0;0;0;0;0;0;0;0;0;0;0;0;0;0;0;0;0;0;0;0;0;0;0;0;0;0;0;0;0;0;0;0;0;0;0;0;0;0;0;0;0;0;0;0;0;0]'}  ClassIndex=1  ClassCtorIndex=1  ClassTabVisible=on  ClassTemplateParamsVisible=off  ClassCtorDeclVisible=on  ClassCtorParamsVisible=on  FunctionTabVisible=on  FunctionDecl=|  PortAttrs={ 'input', 'sig_i', 'adf::input_buffer< cint32, adf::extents< 260 > > & restrict', '260', '0', 'sync', ''; 'output', 'sig_o', 'adf::output_buffer< cint32, adf::extents< 260 > > & restrict', '260', '', 'sync', '' }  PortAttrsEnables={'off', 'off', 'off', 'off', 'off', 'off', 'off';'off', 'off', 'off', 'off', 'off', 'off', 'off'}  SampleTime=-1  ClassDeclTypeOptions=C[1 1]@t16@class ifft256p4;  ClassDecl=class ifft256p4;  ClassTemplateParams={}  ClassTemplateParamsEnables={}  ClassCtorDeclTypeOptions=C[1 1]@t39@ifft256p4(cint32 ( & tbuff_i ) [ 256 ])  ClassCtorDecl=ifft256p4(cint32 ( & tbuff_i ) [ 256 ])  ClassCtorParams={ 'tbuff_i', 'cint32 ( &) [ 256 ]', 'buff_init' }  KernelHeaderFile=aie_src/ifft256p4.h  KernelClassName=ifft256p4  KernelFunction=run  KernelSourceFile=aie_src/ifft256p4.cpp  KernelSearchPaths={}  PreProcOptions={}  blockJsonConstraints=[]
      KernelAllAttrs=|
      | s[12;12;9;9;19;14;21;23;21;23;24;21;15;17;12;24;26;26;26;27;28;9;21;23;23;23;24;25;14;19;19;29]@FunctionNameDeclFileNamePortNamesPortTypesPortSerializedTypesPortDirectionsPortWindowSizeEnablesPortWindowMarginEnablesPortBufferSizeEnablesPortBufferMarginEnablesPortSynchronicityEnablesPortSignalSizeEnablesPortBufferSizesPortBufferMarginsFunctionDeclFunctionTemplateSpecKindFunctionTemplateParamNamesFunctionTemplateParamKindsFunctionTemplateParamTypesFunctionTemplateParamValuesFunctionTemplateParamEnablesClassDeclClassTemplateSpecKindClassTemplateParamNamesClassTemplateParamKindsClassTemplateParamTypesClassTemplateParamValuesClassTemplateParamEnablesClassCtorDeclsClassCtorParamNamesClassCtorParamTypesClassCtorParamSerializedTypes[1 1]@C[32 1]@t3@runt29@../../aie_src/ifft256p4_vmc.hC[2 1]@t5@sig_it5@sig_oC[2 1]@t59@adf::input_buffer< cint32, adf::extents< 260 > > & restrictt60@adf::output_buffer< cint32, adf::extents< 260 > > & restrictC[2 1]@t71@{Q2{R{Tadf::input_buffer{2{t{Scint32}}{t{Tadf::extents{1{t{}260}}}}}}}}t72@{Q2{R{Tadf::output_buffer{2{t{Scint32}}{t{Tadf::extents{1{t{}260}}}}}}}}C[2 1]@t5@inputt6@outputC[2 1]@l1@l1@C[2 1]@l1@l0@C[2 1]@l1@l1@C[2 1]@l0@l0@C[2 1]@l1@l1@C[2 1]@l0@l0@C[2 1]@t3@260t3@260C[2 1]@nnt155@void ifft256p4::
      | run(adf::input_buffer< cint32, adf::extents< 260 > > & restrict sig_i, adf::output_buffer< cint32, adf::extents< 260 > > & restrict sig_o)t4@nonee[0 1]@e[0 1]@e[0 1]@e[0 1]@e[0 1]@t16@class ifft256p4;t4@nonee[0 1]@e[0 1]@e[0 1]@e[0 1]@e[0 1]@C[1 1]@t39@ifft256p4(cint32 ( & tbuff_i ) [ 256 ])C[1 1]@C[1 1]@t7@tbuff_iC[1 1]@C[1 1]@t19@cint32 ( &) [ 256 ]C[1 1]@C[1 1]@t18@{R{C{Scint32}256}}
      FunctionDecl=|
      | void ifft256p4::
      | run(adf::input_buffer< cint32, adf::extents< 260 > > & restrict sig_i, adf::output_buffer< cint32, adf::extents< 260 > > & restrict sig_o)
  ifft256p4_4 : aieBasic/AIE Class Kernel  KernelAllAttrs=|  PortNames={'sig_i'; 'sig_o'}  PortSerializedTypes={'{Q2{R{Tadf::input_buffer{2{t{Scint32}}{t{Tadf::extents{1{t{}260}}}}}}}}'; '{Q2{R{Tadf::output_buffer{2{t{Scint32}}{t{Tadf::extents{1{t{}260}}}}}}}}'}  PortWindowSizes={2.600000000000000000e+02; 2.600000000000000000e+02}  PortWindowMargins={0.000000000000000000e+00; 0.000000000000000000e+00}  PortSynchronicities={'sync', 'sync'}  PortSignalSizes={0.000000000000000000e+00; 0.000000000000000000e+00}  ClassTemplateSpecKind=none  ClassTemplateParamNames={}  ClassTemplateParamKinds={}  ClassTemplateParamTypes={}  ClassTemplateParamValues={}  ClassCtorParamNames={'tbuff_i'}  ClassCtorParamSerializedTypes={'{R{C{Scint32}256}}'}  ClassCtorParamValues={'[0;0;0;0;0;0;0;0;0;0;0;0;0;0;0;0;0;0;0;0;0;0;0;0;0;0;0;0;0;0;0;0;0;0;0;0;0;0;0;0;0;0;0;0;0;0;0;0;0;0;0;0;0;0;0;0;0;0;0;0;0;0;0;0;0;0;0;0;0;0;0;0;0;0;0;0;0;0;0;0;0;0;0;0;0;0;0;0;0;0;0;0;0;0;0;0;0;0;0;0;0;0;0;0;0;0;0;0;0;0;0;0;0;0;0;0;0;0;0;0;0;0;0;0;0;0;0;0;0;0;0;0;0;0;0;0;0;0;0;0;0;0;0;0;0;0;0;0;0;0;0;0;0;0;0;0;0;0;0;0;0;0;0;0;0;0;0;0;0;0;0;0;0;0;0;0;0;0;0;0;0;0;0;0;0;0;0;0;0;0;0;0;0;0;0;0;0;0;0;0;0;0;0;0;0;0;0;0;0;0;0;0;0;0;0;0;0;0;0;0;0;0;0;0;0;0;0;0;0;0;0;0;0;0;0;0;0;0;0;0;0;0;0;0;0;0;0;0;0;0;0;0;0;0;0;0]'}  ClassIndex=1  ClassCtorIndex=1  ClassTabVisible=on  ClassTemplateParamsVisible=off  ClassCtorDeclVisible=on  ClassCtorParamsVisible=on  FunctionTabVisible=on  FunctionDecl=|  PortAttrs={ 'input', 'sig_i', 'adf::input_buffer< cint32, adf::extents< 260 > > & restrict', '260', '0', 'sync', ''; 'output', 'sig_o', 'adf::output_buffer< cint32, adf::extents< 260 > > & restrict', '260', '', 'sync', '' }  PortAttrsEnables={'off', 'off', 'off', 'off', 'off', 'off', 'off';'off', 'off', 'off', 'off', 'off', 'off', 'off'}  SampleTime=-1  ClassDeclTypeOptions=C[1 1]@t16@class ifft256p4;  ClassDecl=class ifft256p4;  ClassTemplateParams={}  ClassTemplateParamsEnables={}  ClassCtorDeclTypeOptions=C[1 1]@t39@ifft256p4(cint32 ( & tbuff_i ) [ 256 ])  ClassCtorDecl=ifft256p4(cint32 ( & tbuff_i ) [ 256 ])  ClassCtorParams={ 'tbuff_i', 'cint32 ( &) [ 256 ]', 'buff_init' }  KernelHeaderFile=aie_src/ifft256p4.h  KernelClassName=ifft256p4  KernelFunction=run  KernelSourceFile=aie_src/ifft256p4.cpp  KernelSearchPaths={}  PreProcOptions={}  blockJsonConstraints=[]
      KernelAllAttrs=|
      | s[12;12;9;9;19;14;21;23;21;23;24;21;15;17;12;24;26;26;26;27;28;9;21;23;23;23;24;25;14;19;19;29]@FunctionNameDeclFileNamePortNamesPortTypesPortSerializedTypesPortDirectionsPortWindowSizeEnablesPortWindowMarginEnablesPortBufferSizeEnablesPortBufferMarginEnablesPortSynchronicityEnablesPortSignalSizeEnablesPortBufferSizesPortBufferMarginsFunctionDeclFunctionTemplateSpecKindFunctionTemplateParamNamesFunctionTemplateParamKindsFunctionTemplateParamTypesFunctionTemplateParamValuesFunctionTemplateParamEnablesClassDeclClassTemplateSpecKindClassTemplateParamNamesClassTemplateParamKindsClassTemplateParamTypesClassTemplateParamValuesClassTemplateParamEnablesClassCtorDeclsClassCtorParamNamesClassCtorParamTypesClassCtorParamSerializedTypes[1 1]@C[32 1]@t3@runt29@../../aie_src/ifft256p4_vmc.hC[2 1]@t5@sig_it5@sig_oC[2 1]@t59@adf::input_buffer< cint32, adf::extents< 260 > > & restrictt60@adf::output_buffer< cint32, adf::extents< 260 > > & restrictC[2 1]@t71@{Q2{R{Tadf::input_buffer{2{t{Scint32}}{t{Tadf::extents{1{t{}260}}}}}}}}t72@{Q2{R{Tadf::output_buffer{2{t{Scint32}}{t{Tadf::extents{1{t{}260}}}}}}}}C[2 1]@t5@inputt6@outputC[2 1]@l1@l1@C[2 1]@l1@l0@C[2 1]@l1@l1@C[2 1]@l0@l0@C[2 1]@l1@l1@C[2 1]@l0@l0@C[2 1]@t3@260t3@260C[2 1]@nnt155@void ifft256p4::
      | run(adf::input_buffer< cint32, adf::extents< 260 > > & restrict sig_i, adf::output_buffer< cint32, adf::extents< 260 > > & restrict sig_o)t4@nonee[0 1]@e[0 1]@e[0 1]@e[0 1]@e[0 1]@t16@class ifft256p4;t4@nonee[0 1]@e[0 1]@e[0 1]@e[0 1]@e[0 1]@C[1 1]@t39@ifft256p4(cint32 ( & tbuff_i ) [ 256 ])C[1 1]@C[1 1]@t7@tbuff_iC[1 1]@C[1 1]@t19@cint32 ( &) [ 256 ]C[1 1]@C[1 1]@t18@{R{C{Scint32}256}}
      FunctionDecl=|
      | void ifft256p4::
      | run(adf::input_buffer< cint32, adf::extents< 260 > > & restrict sig_i, adf::output_buffer< cint32, adf::extents< 260 > > & restrict sig_o)
  Out1 : Outport
  Out2 : Outport  Port=2
  Out3 : Outport  Port=3
  Out4 : Outport  Port=4
  Out5 : Outport  Port=5
  wires:
  In3/1 -> PLIO15/1
  ifft256p4_2/1 -> PLIO16/1
  In1/1 -> PLIO19/1
  ifft256p4_4/1 -> PLIO14/1
  In2/1 -> PLIO11/1
  PLIO9/1 -> Out1/1
  PLIO12/1 -> Out2/1
  In5/1 -> PLIO13/1
  In4/1 -> PLIO17/1
  ifft256p4_1/1 -> PLIO12/1
  PLIO16/1 -> Out3/1
  ifft256p4_3/1 -> PLIO18/1
  ifft256p4_0/1 -> PLIO9/1
  PLIO18/1 -> Out4/1
  PLIO13/1 -> ifft256p4_4/1
  PLIO14/1 -> Out5/1
  PLIO11/1 -> ifft256p4_1/1
  PLIO17/1 -> ifft256p4_3/1
  PLIO15/1 -> ifft256p4_2/1
  PLIO19/1 -> ifft256p4_0/1
